simulink model "modelocontrol"  (R2014a)
settings: Solver=ode45  StartTime=0.0  StopTime=60  FixedStep=0.00001  RelTol=1e-12
values from neighbouring files (symbols this model uses):
  m = [1 t0 (t0)^2 (t0)^3;0 1 (2*(t0)^2) (3*(t0)^2);1 tf (tf)^2 (tf)^3;0 1 (2*(tf)^2) (3*(tf)^2)]    [ControlCinematico.m]    (also in untitled3.m = [1 0 0 0 0 0;0 1 0 0 0 0;0 0 2 0 0 0;1 tf tf^2 tf^3 tf^4 tf^)
libraries: mblibv1 x14
settings Model: Creator=sebastian  LastModifiedBy=root
settings DebuggingCC: UnderspecifiedInitializationDetection=Classic  StateNameClashWarn=warning
settings SimMechanicsCC: VisOnUpdateDiagram=on  VisDuringSimulation=on

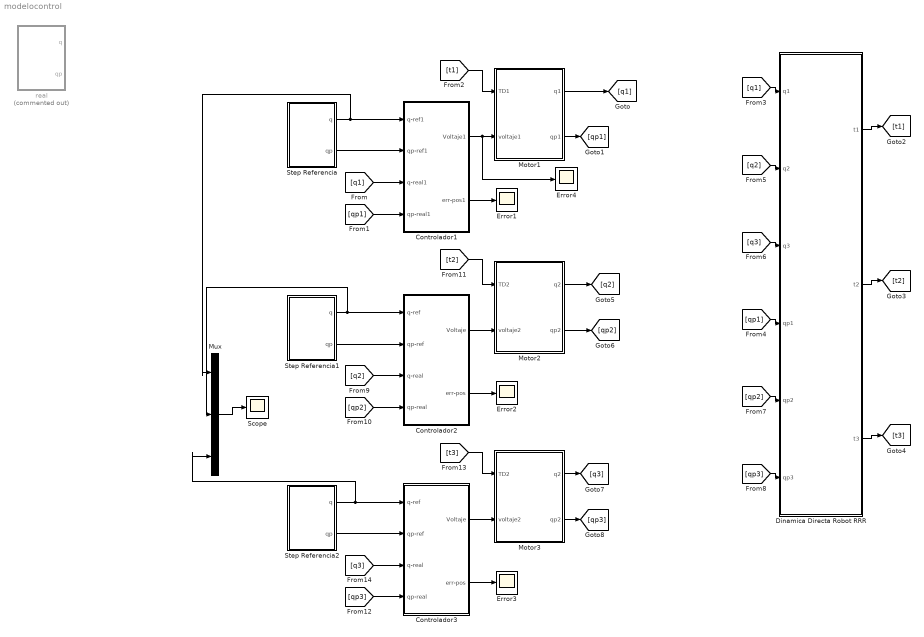
== system modelocontrol ==
  Controlador1 : Subsystem
  Controlador2 : Subsystem
  Controlador3 : Subsystem
  Dinamica Directa Robot RRR : Subsystem
  Error{1..4} (4 alike) : Scope
      Error1 settings: TimeRange=0.000199999999999978  YMin=-470000  YMax=-455000  SaveName=ScopeData4
      Error2 settings: YMin=0.3178  YMax=0.3188
      Error3 settings: YMin=0.675  YMax=1  SaveName=ScopeData5
      Error4 settings: YMin=1.61  YMax=1.73  SaveName=ScopeData12
  Motor1 : Subsystem
  Motor2 : Subsystem
  Motor3 : Subsystem
  Mux : Mux  Inputs=3
  Scope : Scope
      settings: SaveName=ScopeData13
  Step Referencia : Subsystem
  Step Referencia1 : Subsystem
  Step Referencia2 : Subsystem
  real : Subsystem  Commented=on
  wires:
  Controlador1/1(Voltaje1) -> Error4/1, Motor1/2(voltaje1)
  Controlador1/2(err-pos1) -> Error1/1
  Motor1/1(q1) -> [q1]
  Motor1/2(qp1) -> [qp1]
  Dinamica Directa Robot RRR/1(t1) -> [t1]
  [q1] -> Controlador1/3(q-real1)
  [qp1] -> Controlador1/4(qp-real1)
  [q1] -> Dinamica Directa Robot RRR/1(q1)
  [qp1] -> Dinamica Directa Robot RRR/4(qp1)
  [q2] -> Dinamica Directa Robot RRR/2(q2)
  [q3] -> Dinamica Directa Robot RRR/3(q3)
  [qp2] -> Dinamica Directa Robot RRR/5(qp2)
  [qp3] -> Dinamica Directa Robot RRR/6(qp3)
  Dinamica Directa Robot RRR/2(t2) -> [t2]
  Dinamica Directa Robot RRR/3(t3) -> [t3]
  Step Referencia1/1(q) -> Mux/2, Controlador2/1(q-ref)
  Step Referencia1/2(qp) -> Controlador2/2(qp-ref)
  Controlador2/1(Voltaje) -> Motor2/2(voltaje2)
  Controlador2/2(err-pos) -> Error2/1
  [q2] -> Controlador2/3(q-real)
  [qp2] -> Controlador2/4(qp-real)
  Step Referencia/1(q) -> Mux/1, Controlador1/1(q-ref1)
  Step Referencia/2(qp) -> Controlador1/2(qp-ref1)
  Step Referencia2/1(q) -> Mux/3, Controlador3/1(q-ref)
  Step Referencia2/2(qp) -> Controlador3/2(qp-ref)
  Controlador3/1(Voltaje) -> Motor3/2(voltaje2)
  Controlador3/2(err-pos) -> Error3/1
  Motor3/1(q2) -> [q3]
  Motor3/2(qp2) -> [qp3]
  [q3] -> Controlador3/3(q-real)
  [qp3] -> Controlador3/4(qp-real)
  Motor2/1(q2) -> [q2]
  Motor2/2(qp2) -> [qp2]
  [t1] -> Motor1/1(TD1)
  [t2] -> Motor2/1(TD2)
  [t3] -> Motor3/1(TD2)
  Mux/1 -> Scope/1

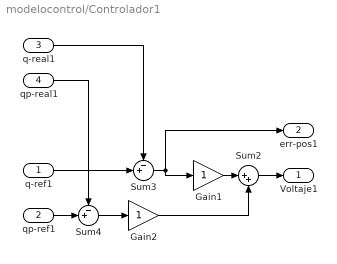
== system modelocontrol/Controlador1 ==
  q-ref1 : Inport
  qp-ref1 : Inport  Port=2
  q-real1 : Inport  Port=3
  qp-real1 : Inport  Port=4
  Gain1 : Gain
  Gain2 : Gain
  Sum2 : Sum  Inputs=|++
  Sum3 : Sum  Inputs=-+|
  Sum4 : Sum  Inputs=-+|
  Voltaje1 : Outport
  err-pos1 : Outport  Port=2
  wires:
  Gain1/1 -> Sum2/1
  Gain2/1 -> Sum2/2
  Sum4/1 -> Gain2/1
  Sum2/1 -> Voltaje1/1
  q-ref1/1 -> Sum3/2
  qp-ref1/1 -> Sum4/2
  q-real1/1 -> Sum3/1
  qp-real1/1 -> Sum4/1
  Sum3/1 -> Gain1/1, err-pos1/1

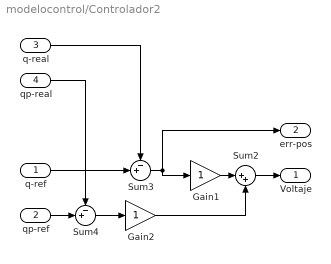
== system modelocontrol/Controlador2 ==
  q-ref : Inport
  qp-ref : Inport  Port=2
  q-real : Inport  Port=3
  qp-real : Inport  Port=4
  Gain1 : Gain
  Gain2 : Gain
  Sum2 : Sum  Inputs=|++
  Sum3 : Sum  Inputs=-+|
  Sum4 : Sum  Inputs=-+|
  Voltaje : Outport
  err-pos : Outport  Port=2
  wires:
  Gain1/1 -> Sum2/1
  Gain2/1 -> Sum2/2
  Sum4/1 -> Gain2/1
  Sum2/1 -> Voltaje/1
  q-ref/1 -> Sum3/2
  qp-ref/1 -> Sum4/2
  q-real/1 -> Sum3/1
  qp-real/1 -> Sum4/1
  Sum3/1 -> Gain1/1, err-pos/1

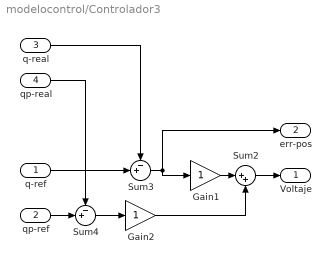
== system modelocontrol/Controlador3 ==
  q-ref : Inport
  qp-ref : Inport  Port=2
  q-real : Inport  Port=3
  qp-real : Inport  Port=4
  Gain1 : Gain
  Gain2 : Gain
  Sum2 : Sum  Inputs=|++
  Sum3 : Sum  Inputs=-+|
  Sum4 : Sum  Inputs=-+|
  Voltaje : Outport
  err-pos : Outport  Port=2
  wires:
  Gain1/1 -> Sum2/1
  Gain2/1 -> Sum2/2
  Sum4/1 -> Gain2/1
  Sum2/1 -> Voltaje/1
  q-ref/1 -> Sum3/2
  qp-ref/1 -> Sum4/2
  q-real/1 -> Sum3/1
  qp-real/1 -> Sum4/1
  Sum3/1 -> Gain1/1, err-pos/1

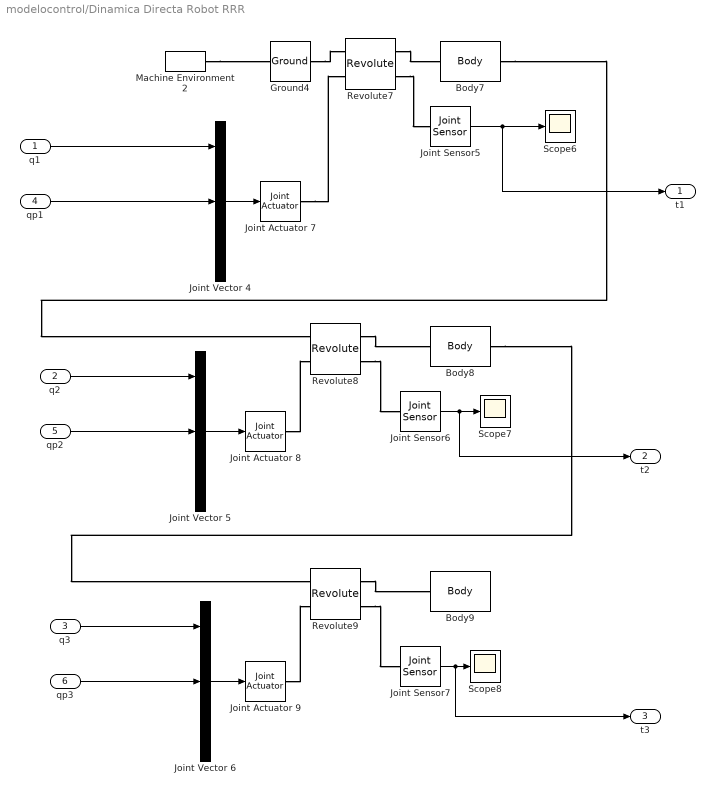
== system modelocontrol/Dinamica Directa Robot RRR ==
  q1 : Inport
  q2 : Inport  Port=2
  q3 : Inport  Port=3
  qp1 : Inport  Port=4
  qp2 : Inport  Port=5
  qp3 : Inport  Port=6
  Body7 : mblibv1/Bodies/Body  LConnTagsString=CS1  RConnTagsString=CS2  UpdateFromCAD=off  DialogClass=MechanicalBodyBlock  Mass=1  MassUnits=kg  InertiaUnits=kg*m^2  Inertia=[0 0 0;0 0 0;0 0 33.3333]  Shape=Cylinder  ShapeDims=[1 1]  ShapeUnits=m  ShapeUse=false  Density=1  DensityUnits=kg/m^3  DensityUse=false  GraphicsMode=MACHINE_DEFAULT  BodyColorSelMode=COLORPALETTE  BodyColor=[0;1;0]  AttachedToCS=CG  CG=Left$CG$[10 0 0]$WORLD$WORLD$m$[0 0 0]$Euler X-Y-Z$deg$WORLD$false$none  WorkingFrames=Left$CS1$[0 0 0]$World$World$m$[0 0 0]$Euler X-Y-Z$deg$WORLD$true$none#Right$CS2$[20 0 0]$World$World$m$[0 0 0]$Euler X-Y-Z$deg$WORLD$true$none  CGPos=[10 0 0]  CGRot=[0 0 0]  CS0Pos=[]  CS0Rot=[]  CS1Pos=[0 0 0]  CS1Rot=[0 0 0]  CS2Pos=[20 0 0]  CS2Rot=[0 0 0]  CS3Pos=[]  CS3Rot=[]  CS4Pos=[]  CS4Rot=[]  CS5Pos=[]  CS5Rot=[]  CS6Pos=[]  CS6Rot=[]  CS7Pos=[]  CS7Rot=[]  CS8Pos=[]  CS8Rot=[]  CS9Pos=[]  CS9Rot=[]  CS10Pos=[]  CS10Rot=[]  CS11Pos=[]  CS11Rot=[]  CS12Pos=[]  CS12Rot=[]  CS13Pos=[]  CS13Rot=[]  CS14Pos=[]  CS14Rot=[]  CS15Pos=[]  CS15Rot=[]  CS16Pos=[]  CS16Rot=[]  CS17Pos=[]  CS17Rot=[]  CS18Pos=[]  CS18Rot=[]  CS19Pos=[]  CS19Rot=[]  CS20Pos=[]  CS20Rot=[]
  Body8 : mblibv1/Bodies/Body  LConnTagsString=CS1  RConnTagsString=CS2  UpdateFromCAD=off  DialogClass=MechanicalBodyBlock  Mass=1  MassUnits=kg  InertiaUnits=kg*m^2  Inertia=[0 0 0;0 0 0;0 0 33.3333]  Shape=Cylinder  ShapeDims=[1 1]  ShapeUnits=m  ShapeUse=false  Density=1  DensityUnits=kg/m^3  DensityUse=false  GraphicsMode=MACHINE_DEFAULT  BodyColorSelMode=COLORPALETTE  BodyColor=[0;1;0]  AttachedToCS=CG  CG=Left$CG$[30 0 0]$WORLD$WORLD$m$[0 0 0]$Euler X-Y-Z$deg$WORLD$false$none  WorkingFrames=Left$CS1$[20 0 0]$World$World$m$[0 0 0]$Euler X-Y-Z$deg$WORLD$true$none#Right$CS2$[40 0 0]$World$World$m$[0 0 0]$Euler X-Y-Z$deg$WORLD$true$none  CGPos=[30 0 0]  CGRot=[0 0 0]  CS0Pos=[]  CS0Rot=[]  CS1Pos=[20 0 0]  CS1Rot=[0 0 0]  CS2Pos=[40 0 0]  CS2Rot=[0 0 0]  CS3Pos=[]  CS3Rot=[]  CS4Pos=[]  CS4Rot=[]  CS5Pos=[]  CS5Rot=[]  CS6Pos=[]  CS6Rot=[]  CS7Pos=[]  CS7Rot=[]  CS8Pos=[]  CS8Rot=[]  CS9Pos=[]  CS9Rot=[]  CS10Pos=[]  CS10Rot=[]  CS11Pos=[]  CS11Rot=[]  CS12Pos=[]  CS12Rot=[]  CS13Pos=[]  CS13Rot=[]  CS14Pos=[]  CS14Rot=[]  CS15Pos=[]  CS15Rot=[]  CS16Pos=[]  CS16Rot=[]  CS17Pos=[]  CS17Rot=[]  CS18Pos=[]  CS18Rot=[]  CS19Pos=[]  CS19Rot=[]  CS20Pos=[]  CS20Rot=[]
  Body9 : mblibv1/Bodies/Body  LConnTagsString=CS1  RConnTagsString=CS2  UpdateFromCAD=off  DialogClass=MechanicalBodyBlock  Mass=1  MassUnits=kg  InertiaUnits=kg*m^2  Inertia=[0 0 0;0 0 0;0 0 8.3333]  Shape=Cylinder  ShapeDims=[1 1]  ShapeUnits=m  ShapeUse=false  Density=1  DensityUnits=kg/m^3  DensityUse=false  GraphicsMode=MACHINE_DEFAULT  BodyColorSelMode=COLORPALETTE  BodyColor=[0;1;0]  AttachedToCS=CG  CG=Left$CG$[45 0 0]$WORLD$WORLD$m$[0 0 0]$Euler X-Y-Z$deg$WORLD$false$none  WorkingFrames=Left$CS1$[40 0 0]$World$World$m$[0 0 0]$Euler X-Y-Z$deg$WORLD$true$none#Right$CS2$[50 0 0]$World$World$m$[0 0 0]$Euler X-Y-Z$deg$WORLD$true$none  CGPos=[45 0 0]  CGRot=[0 0 0]  CS0Pos=[]  CS0Rot=[]  CS1Pos=[40 0 0]  CS1Rot=[0 0 0]  CS2Pos=[50 0 0]  CS2Rot=[0 0 0]  CS3Pos=[]  CS3Rot=[]  CS4Pos=[]  CS4Rot=[]  CS5Pos=[]  CS5Rot=[]  CS6Pos=[]  CS6Rot=[]  CS7Pos=[]  CS7Rot=[]  CS8Pos=[]  CS8Rot=[]  CS9Pos=[]  CS9Rot=[]  CS10Pos=[]  CS10Rot=[]  CS11Pos=[]  CS11Rot=[]  CS12Pos=[]  CS12Rot=[]  CS13Pos=[]  CS13Rot=[]  CS14Pos=[]  CS14Rot=[]  CS15Pos=[]  CS15Rot=[]  CS16Pos=[]  CS16Rot=[]  CS17Pos=[]  CS17Rot=[]  CS18Pos=[]  CS18Rot=[]  CS19Pos=[]  CS19Rot=[]  CS20Pos=[]  CS20Rot=[]
  Ground4 : mblibv1/Bodies/Ground  UpdateFromCAD=off  LeftPortType=env  RightPortType=workingframe  PhysicalDomain=Mechanical  DialogClass=GroundBlock  CoordPosition=[0 0 0]  CoordPositionUnits=m  StateVectorMgrId=2  MachineId=[3 0]  ShowEnvPort=on  ParameterChecksum=[2542761875, 2426724538, 2990906651, 1146370268]  TopologyChecksum=[2378030560, 2017794222, 1685964279, 1068232264]
  Joint Actuator 7 : mblibv1/Sensors &  Actuators/Joint Actuator  UpdateFromCAD=off  PhysicalDomain=Mechanical  PortType=blob  ActuationStyle=Motion  AngleUnits=rad  ArcVelocityUnits=rad/s  ArcAccelerationUnits=rad/s^2  CoordPositionUnits=m  VelocityUnits=m/s  AccelerationUnits=m/s^2  ForceUnits=N  TorqueUnits=N*m  ActiveIO=on  Width=3  DialogClass=MechanicalActuatorBlock  Primitive=R1  ReferenceFrame=Absolute (World)
  Joint Actuator 8 : mblibv1/Sensors &  Actuators/Joint Actuator  UpdateFromCAD=off  PhysicalDomain=Mechanical  PortType=blob  ActuationStyle=Motion  AngleUnits=rad  ArcVelocityUnits=rad/s  ArcAccelerationUnits=rad/s^2  CoordPositionUnits=m  VelocityUnits=m/s  AccelerationUnits=m/s^2  ForceUnits=N  TorqueUnits=N*m  ActiveIO=on  Width=3  DialogClass=MechanicalActuatorBlock  Primitive=R1  ReferenceFrame=Absolute (World)
  Joint Actuator 9 : mblibv1/Sensors &  Actuators/Joint Actuator  UpdateFromCAD=off  PhysicalDomain=Mechanical  PortType=blob  ActuationStyle=Motion  AngleUnits=rad  ArcVelocityUnits=rad/s  ArcAccelerationUnits=rad/s^2  CoordPositionUnits=m  VelocityUnits=m/s  AccelerationUnits=m/s^2  ForceUnits=N  TorqueUnits=N*m  ActiveIO=on  Width=3  DialogClass=MechanicalActuatorBlock  Primitive=R1  ReferenceFrame=Absolute (World)
  Joint Sensor5 : mblibv1/Sensors &  Actuators/Joint Sensor  UpdateFromCAD=off  PhysicalDomain=Mechanical  PortType=blob  Muxed=on  Pose=off  Angle=off  AngleUnits=deg  ArcVelocity=off  ArcVelocityUnits=deg/s  ArcAcceleration=off  ArcAccelerationUnits=deg/s^2  CoordPosition=on  CoordPositionUnits=m  Velocity=off  VelocityUnits=m/s  Acceleration=off  AccelerationUnits=m/s^2  Quaternion=on  QuaternionDT=off  QuaternionDDT=off  QuaternionUnits=off  OutputVector=[1]  ActiveIO=on  Width=1  DialogClass=MechanicalSensorBlock  Primitive=R1  Force=off  ForceUnits=N  Torque=on  TorqueUnits=N*m  ReferenceFrame=Absolute (World)  ReactionSensedSide=Follower  ReactionReferenceFrame=Absolute (World)  ReactionForce=off  ReactionForceUnits=N  ReactionMoment=off  ReactionMomentUnits=N*m
  Joint Sensor6 : mblibv1/Sensors &  Actuators/Joint Sensor  UpdateFromCAD=off  PhysicalDomain=Mechanical  PortType=blob  Muxed=on  Pose=off  Angle=off  AngleUnits=deg  ArcVelocity=off  ArcVelocityUnits=deg/s  ArcAcceleration=off  ArcAccelerationUnits=deg/s^2  CoordPosition=on  CoordPositionUnits=m  Velocity=off  VelocityUnits=m/s  Acceleration=off  AccelerationUnits=m/s^2  Quaternion=on  QuaternionDT=off  QuaternionDDT=off  QuaternionUnits=off  OutputVector=[1]  ActiveIO=on  Width=1  DialogClass=MechanicalSensorBlock  Primitive=R1  Force=off  ForceUnits=N  Torque=on  TorqueUnits=N*m  ReferenceFrame=Absolute (World)  ReactionSensedSide=Follower  ReactionReferenceFrame=Absolute (World)  ReactionForce=off  ReactionForceUnits=N  ReactionMoment=off  ReactionMomentUnits=N*m
  Joint Sensor7 : mblibv1/Sensors &  Actuators/Joint Sensor  UpdateFromCAD=off  PhysicalDomain=Mechanical  PortType=blob  Muxed=on  Pose=off  Angle=off  AngleUnits=deg  ArcVelocity=off  ArcVelocityUnits=deg/s  ArcAcceleration=off  ArcAccelerationUnits=deg/s^2  CoordPosition=on  CoordPositionUnits=m  Velocity=off  VelocityUnits=m/s  Acceleration=off  AccelerationUnits=m/s^2  Quaternion=on  QuaternionDT=off  QuaternionDDT=off  QuaternionUnits=off  OutputVector=[1]  ActiveIO=on  Width=1  DialogClass=MechanicalSensorBlock  Primitive=R1  Force=off  ForceUnits=N  Torque=on  TorqueUnits=N*m  ReferenceFrame=Absolute (World)  ReactionSensedSide=Follower  ReactionReferenceFrame=Absolute (World)  ReactionForce=off  ReactionForceUnits=N  ReactionMoment=off  ReactionMomentUnits=N*m
  Joint Vector 4 : Concatenate  NumInputs=3
  Joint Vector 5 : Concatenate  NumInputs=3
  Joint Vector 6 : Concatenate  NumInputs=3
  Machine Environment2 : mblibv1/Bodies/Machine Environment  PortType=env  PhysicalDomain=Mechanical  DialogTemplateClass=MECH.MachineEnvironment  SyncWhenCopied=off  Gravity=[0 0 0]  GravityUnits=m/s^2  GravityAsSignal=off  Dimensionality=Auto-detect  AnalysisType=Inverse dynamics  LinearAssemblyTolerance=1e-3  LinearAssemblyToleranceUnits=m  AngularAssemblyTolerance=1e-3  AngularAssemblyToleranceUnits=rad  ConstraintSolverType=Stabilizing  ConstraintRelTolerance=1e-4  ConstraintAbsTolerance=1e-4  UseRobustSingularityHandling=off  RedundancyAnalysisToleranceType=Automatically select tolerance  RedundancyAnalysisTolerance=1e-14  StatePerturbationType=Fixed  PerturbationSize=1e-5  VisualizeMachine=on  BodyVisualizationType=Use model default body geometries  BodyColorSelMode=Use model default  DefaultBodyColor=[1 0 0]
  Revolute7 : mblibv1/Joints/Revolute  LConnTagsString=__newl0|SA1  RConnTagsString=__newr0|SA1  UpdateFromCAD=off  NumSAPorts=2  CutJoint=off  MarkAsCut=off  Primitives=prismatic  PrimitiveProps=R1$World$[0 0 1]$revolute  DialogClass=JointBlock  R1Axis=[0 0 1]
  Revolute8 : mblibv1/Joints/Revolute  LConnTagsString=__newl0|SA1  RConnTagsString=__newr0|SA1  UpdateFromCAD=off  NumSAPorts=2  CutJoint=off  MarkAsCut=off  Primitives=prismatic  PrimitiveProps=R1$World$[0 0 1]$revolute  DialogClass=JointBlock  R1Axis=[0 0 1]
  Revolute9 : mblibv1/Joints/Revolute  LConnTagsString=__newl0|SA1  RConnTagsString=__newr0|SA1  UpdateFromCAD=off  NumSAPorts=2  CutJoint=off  MarkAsCut=off  Primitives=prismatic  PrimitiveProps=R1$World$[0 0 1]$revolute  DialogClass=JointBlock  R1Axis=[0 0 1]
  Scope6 : Scope
      settings: TimeRange=30  YMin=-2.525e+08  YMax=-2.35e+08  SaveName=ScopeData9
  Scope7 : Scope
      settings: TimeRange=30  SaveName=ScopeData10
  Scope8 : Scope
      settings: TimeRange=30  SaveName=ScopeData11
  t1 : Outport
  t2 : Outport  Port=2
  t3 : Outport  Port=3
  wires:
  Joint Vector 5/1 -> Joint Actuator 8/1
  Joint Vector 4/1 -> Joint Actuator 7/1
  Joint Vector 6/1 -> Joint Actuator 9/1
  Joint Sensor5/1 -> t1/1, Scope6/1
  Joint Sensor7/1 -> t3/1, Scope8/1
  Joint Sensor6/1 -> t2/1, Scope7/1
  q1/1 -> Joint Vector 4/1
  q2/1 -> Joint Vector 5/1
  q3/1 -> Joint Vector 6/1
  qp1/1 -> Joint Vector 4/2
  qp2/1 -> Joint Vector 5/2
  qp3/1 -> Joint Vector 6/2
  connections:
  Revolute9/RConn1 -- Body9/LConn1
  Body7/RConn1 -- Revolute8/LConn1
  Body8/RConn1 -- Revolute9/LConn1
  Revolute8/RConn2 -- Joint Sensor6/LConn1
  Joint Actuator 8/RConn1 -- Revolute8/LConn2
  Revolute8/RConn1 -- Body8/LConn1
  Ground4/RConn1 -- Revolute7/LConn1
  Revolute7/RConn1 -- Body7/LConn1
  Revolute7/RConn2 -- Joint Sensor5/LConn1
  Revolute9/RConn2 -- Joint Sensor7/LConn1
  Joint Actuator 9/RConn1 -- Revolute9/LConn2
  Machine Environment2/RConn1 -- Ground4/LConn1
  Joint Actuator 7/RConn1 -- Revolute7/LConn2

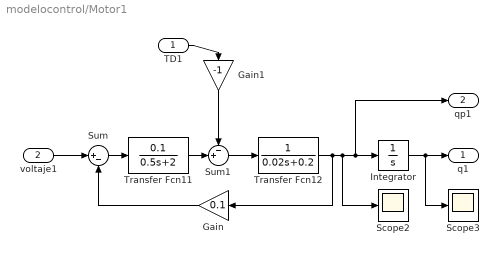
== system modelocontrol/Motor1 ==
  TD1 : Inport
  voltaje1 : Inport  Port=2
  Gain : Gain  Gain=0.1
  Gain1 : Gain  Gain=-1
  Integrator : Integrator
  Scope2 : Scope
  Scope3 : Scope
      settings: SaveName=ScopeData3
  Sum : Sum  Inputs=|+-
  Sum1 : Sum  Inputs=-+|
  Transfer Fcn11 : TransferFcn  Numerator=[0.1]  Denominator=[0.5 2]
  Transfer Fcn12 : TransferFcn  Denominator=[0.02 0.2]
  q1 : Outport
  qp1 : Outport  Port=2
  wires:
  Sum/1 -> Transfer Fcn11/1
  Sum1/1 -> Transfer Fcn12/1
  Transfer Fcn11/1 -> Sum1/2
  Gain/1 -> Sum/2
  Transfer Fcn12/1 -> qp1/1, Integrator/1, Scope2/1, Gain/1
  Integrator/1 -> q1/1, Scope3/1
  voltaje1/1 -> Sum/1
  TD1/1 -> Gain1/1
  Gain1/1 -> Sum1/1

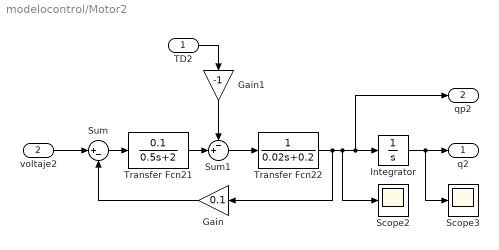
== system modelocontrol/Motor2 ==
  TD2 : Inport
  voltaje2 : Inport  Port=2
  Gain : Gain  Gain=0.1
  Gain1 : Gain  Gain=-1
  Integrator : Integrator
  Scope2 : Scope
  Scope3 : Scope
      settings: SaveName=ScopeData3
  Sum : Sum  Inputs=|+-
  Sum1 : Sum  Inputs=-+|
  Transfer Fcn21 : TransferFcn  Numerator=[0.1]  Denominator=[0.5 2]
  Transfer Fcn22 : TransferFcn  Denominator=[0.02 0.2]
  q2 : Outport
  qp2 : Outport  Port=2
  wires:
  Sum/1 -> Transfer Fcn21/1
  Sum1/1 -> Transfer Fcn22/1
  Transfer Fcn21/1 -> Sum1/2
  Gain/1 -> Sum/2
  Transfer Fcn22/1 -> qp2/1, Integrator/1, Scope2/1, Gain/1
  Integrator/1 -> q2/1, Scope3/1
  voltaje2/1 -> Sum/1
  TD2/1 -> Gain1/1
  Gain1/1 -> Sum1/1

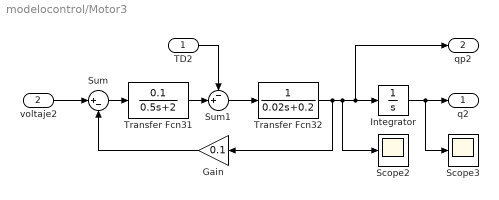
== system modelocontrol/Motor3 ==
  TD2 : Inport
  voltaje2 : Inport  Port=2
  Gain : Gain  Gain=0.1
  Integrator : Integrator
  Scope2 : Scope
  Scope3 : Scope
      settings: SaveName=ScopeData3
  Sum : Sum  Inputs=|+-
  Sum1 : Sum  Inputs=-+|
  Transfer Fcn31 : TransferFcn  Numerator=[0.1]  Denominator=[0.5 2]
  Transfer Fcn32 : TransferFcn  Denominator=[0.02 0.2]
  q2 : Outport
  qp2 : Outport  Port=2
  wires:
  Sum/1 -> Transfer Fcn31/1
  Sum1/1 -> Transfer Fcn32/1
  Transfer Fcn31/1 -> Sum1/2
  Gain/1 -> Sum/2
  Transfer Fcn32/1 -> qp2/1, Integrator/1, Scope2/1, Gain/1
  Integrator/1 -> q2/1, Scope3/1
  voltaje2/1 -> Sum/1
  TD2/1 -> Sum1/1

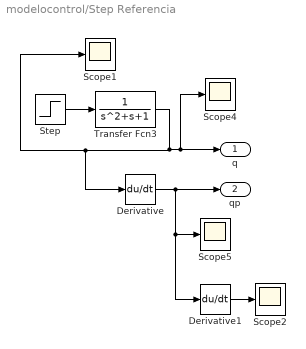
== system modelocontrol/Step Referencia ==
  Derivative : Derivative
  Derivative1 : Derivative
  Scope{1..2,4..5} (4 alike) : Scope
      Scope1 settings: SaveName=ScopeData6
      Scope2 settings: SaveName=ScopeData2
      Scope4 settings: SaveName=ScopeData7
      Scope5 settings: SaveName=ScopeData8
  Step : Step  After=0.1  SampleTime=0
  Transfer Fcn3 : TransferFcn  Denominator=[1 1 1]
  q : Outport
  qp : Outport  Port=2
  wires:
  Step/1 -> Transfer Fcn3/1
  Transfer Fcn3/1 -> q/1, Scope4/1, Derivative/1, Scope1/1
  Derivative/1 -> Derivative1/1, Scope5/1, qp/1
  Derivative1/1 -> Scope2/1

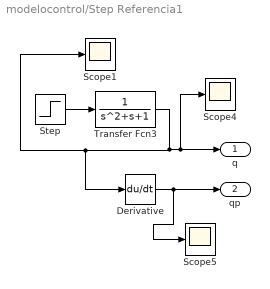
== system modelocontrol/Step Referencia1 ==
  Derivative : Derivative
  Scope1 : Scope
      settings: SaveName=ScopeData6
  Scope4 : Scope
      settings: SaveName=ScopeData7
  Scope5 : Scope
      settings: SaveName=ScopeData8
  Step : Step  After=0.1  SampleTime=0
  Transfer Fcn3 : TransferFcn  Denominator=[1 1 1]
  q : Outport
  qp : Outport  Port=2
  wires:
  Step/1 -> Transfer Fcn3/1
  Transfer Fcn3/1 -> q/1, Scope4/1, Derivative/1, Scope1/1
  Derivative/1 -> Scope5/1, qp/1

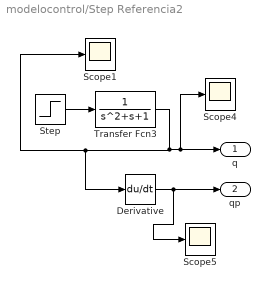
== system modelocontrol/Step Referencia2 ==
  Derivative : Derivative
  Scope1 : Scope
      settings: SaveName=ScopeData6
  Scope4 : Scope
      settings: SaveName=ScopeData7
  Scope5 : Scope
      settings: SaveName=ScopeData8
  Step : Step  After=0.1  SampleTime=0
  Transfer Fcn3 : TransferFcn  Denominator=[1 1 1]
  q : Outport
  qp : Outport  Port=2
  wires:
  Step/1 -> Transfer Fcn3/1
  Transfer Fcn3/1 -> q/1, Scope4/1, Derivative/1, Scope1/1
  Derivative/1 -> Scope5/1, qp/1

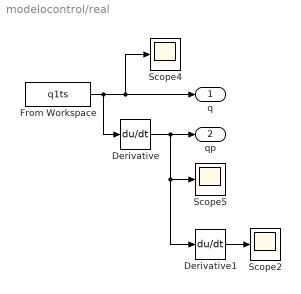
== system modelocontrol/real ==
  Derivative : Derivative
  Derivative1 : Derivative
  From Workspace : FromWorkspace  VariableName=q1ts  SampleTime=0  OutputAfterFinalValue=Holding final value
  Scope2 : Scope
      settings: SaveName=ScopeData2
  Scope4 : Scope
      settings: SaveName=ScopeData7
  Scope5 : Scope
      settings: SaveName=ScopeData8
  q : Outport
  qp : Outport  Port=2
  wires:
  Derivative/1 -> Derivative1/1, Scope5/1, qp/1
  Derivative1/1 -> Scope2/1
  From Workspace/1 -> Derivative/1, Scope4/1, q/1
